simulink model "zad2"  (R2017a)
settings: Solver=VariableStepAuto  StartTime=0.0  StopTime=16  RelTol=1e-3
settings Model: Creator=DoktorHax  LastModifiedBy=DoktorHax

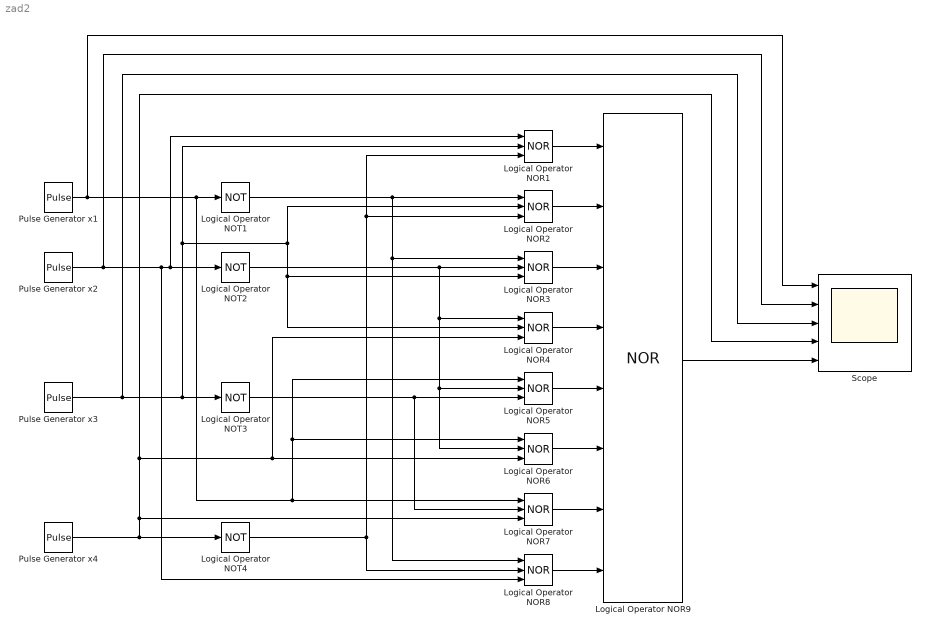
== system zad2 ==
  Logical Operator NOR{1..8} (8 alike) : Logic  Operator=NOR  Inputs=3  AllPortsSameDT=off  OutDataTypeStr=boolean
  Logical Operator NOR9 : Logic  Operator=NOR  Inputs=8  AllPortsSameDT=off  OutDataTypeStr=boolean
  Logical Operator NOT{1..4} (4 alike) : Logic  Operator=NOT  AllPortsSameDT=off  OutDataTypeStr=boolean
  Pulse Generator x1 : DiscretePulseGenerator  PulseType=Time based  PulseWidth=50
  Pulse Generator x2 : DiscretePulseGenerator  PulseType=Time based  Period=4  PulseWidth=50
  Pulse Generator x3 : DiscretePulseGenerator  PulseType=Time based  Period=8  PulseWidth=50
  Pulse Generator x4 : DiscretePulseGenerator  PulseType=Time based  Period=16  PulseWidth=50
  Scope : Scope  NumInputPorts=5
  wires:
  Logical Operator NOR1/1 -> Logical Operator NOR9/1
  Logical Operator NOR9/1 -> Scope/5
  Logical Operator NOR2/1 -> Logical Operator NOR9/2
  Logical Operator NOR3/1 -> Logical Operator NOR9/3
  Logical Operator NOR4/1 -> Logical Operator NOR9/4
  Logical Operator NOR5/1 -> Logical Operator NOR9/5
  Logical Operator NOR6/1 -> Logical Operator NOR9/6
  Logical Operator NOR7/1 -> Logical Operator NOR9/7
  Pulse Generator x4/1 -> Scope/4, Logical Operator NOR4/3, Logical Operator NOR6/3, Logical Operator NOR7/3, Logical Operator NOT4/1
  Pulse Generator x3/1 -> Scope/3, Logical Operator NOR4/2, Logical Operator NOR3/3, Logical Operator NOR2/2, Logical Operator NOR1/2, Logical Operator NOT3/1
  Pulse Generator x2/1 -> Scope/2, Logical Operator NOR1/1, Logical Operator NOT2/1, Logical Operator NOR8/3
  Pulse Generator x1/1 -> Scope/1, Logical Operator NOR7/1, Logical Operator NOR6/1, Logical Operator NOR5/1, Logical Operator NOT1/1
  Logical Operator NOT4/1 -> Logical Operator NOR8/2, Logical Operator NOR2/3, Logical Operator NOR1/3
  Logical Operator NOT1/1 -> Logical Operator NOR2/1, Logical Operator NOR3/1, Logical Operator NOR8/1
  Logical Operator NOT2/1 -> Logical Operator NOR4/1, Logical Operator NOR5/2, Logical Operator NOR6/2, Logical Operator NOR3/2
  Logical Operator NOT3/1 -> Logical Operator NOR5/3, Logical Operator NOR7/2
  Logical Operator NOR8/1 -> Logical Operator NOR9/8
